simulink model "scars_example_appendix"  (R2019b)
settings: Solver=ode14x  StartTime=0.0  StopTime=300  FixedStep=0.1  RelTol=1e-3
libraries: scars_library x7
settings Model: Creator=asmialek  LastModifiedBy=asmialek
settings DataIOCC: ReturnWorkspaceOutputsName=scars_out

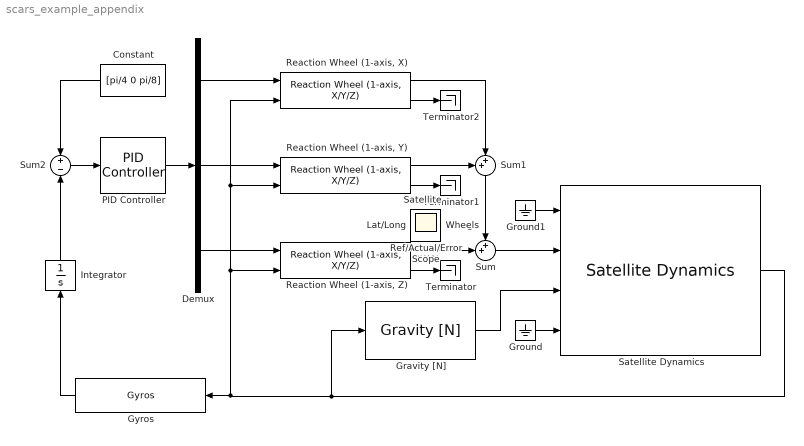
== system scars_example_appendix ==
  " Satellite Dynamics " : scars_library/Standard/ Satellite Dynamics   Parameter4=Keplerian Elements  epoch=0  mass=0  a=6356e3+400e3  e=0  incl=0  RA=0  w=0  TA=0  initEuler=[0 0 0]  initEulerRates=[0 0 0]  TA_copy=0  TA_copy_copy=400e3  TA_copy_copy_copy=[10 25]  TA_copy_copy_copy_copy=[10 25]  initEuler_copy=[0 0 0]  initEulerRates_copy=[0 0 0]  SSRTWFcnClass=[]
  Constant : Constant  Value=[pi/4 0 pi/8]
  Demux : Demux  Outputs=3
  Gravity [N] : scars_library/Environment/Gravity [N]  mass=1
  Ground : Ground
  Ground1 : Ground
  Gyros : scars_library/Sensors/Gyros  g_wn=14500  g_zeta=sqrt(2)/2  g_freq=10  g_bias=0  g_power=(2*pi*0.04/360)^2  g_max=deg2rad(75)  g_min=-deg2rad(75)
  Integrator : Integrator  InitialCondition=[0.76 2.32 1.71]
  PID Controller : scars_library/ Control Algorithms /PID Controller  Kp=700  Ki=0.01  Kd=1000  pid_sat_max=inf  pid_sat_min=-inf  pid_dz_max=0  pid_dz_min=0
  "Reaction Wheel (1-axis, X)" : scars_library/Actuators/Reaction Wheel (1-axis, X//Y//Z)  axis_switch=X  N=(1.5e-3)/0.5  R=12  J=300e-3  c=0  vel_max=6000*2*pi/60  torq_max=1.5e-3  i_max=0.5  rw_power=0  rw_freq=0.1
  "Reaction Wheel (1-axis, Y)" : scars_library/Actuators/Reaction Wheel (1-axis, X//Y//Z)  axis_switch=Y  N=(1.5e-3)/0.5  R=12  J=300e-3  c=0  vel_max=6000*2*pi/60  torq_max=1.5e-3  i_max=0.5  rw_power=0  rw_freq=0.1
  "Reaction Wheel (1-axis, Z)" : scars_library/Actuators/Reaction Wheel (1-axis, X//Y//Z)  axis_switch=Z  N=(1.5e-3)/0.5  R=12  J=300e-3  c=0  vel_max=6000*2*pi/60  torq_max=1.5e-3  i_max=0.5  rw_power=0  rw_freq=0.1
  Sum : Sum  Inputs=++|
  Sum1 : Sum  Inputs=++|
  Sum2 : Sum  Inputs=+|-
  Terminator : Terminator
  Terminator1 : Terminator
  Terminator2 : Terminator
  Lat/Long : Scope
  Omega : Scope
  RW Y : Scope
  Ref/Actual/Error : Scope
  Satellite : Scope
  Scope : Scope
  Wheels : Scope
  wires:
  Ground/1 -> " Satellite Dynamics "/4
  Gravity [N]/1 -> " Satellite Dynamics "/3
  " Satellite Dynamics "/1 -> Gravity [N]/1, "Reaction Wheel (1-axis, X)"/2, "Reaction Wheel (1-axis, Y)"/2, "Reaction Wheel (1-axis, Z)"/2, Gyros/1
  Ground1/1 -> " Satellite Dynamics "/1
  "Reaction Wheel (1-axis, Z)"/1 -> Sum/2
  "Reaction Wheel (1-axis, Z)"/2 -> Terminator/1
  "Reaction Wheel (1-axis, Y)"/2 -> Terminator1/1
  "Reaction Wheel (1-axis, X)"/2 -> Terminator2/1
  Sum/1 -> " Satellite Dynamics "/2
  "Reaction Wheel (1-axis, Y)"/1 -> Sum1/1
  Sum1/1 -> Sum/1
  "Reaction Wheel (1-axis, X)"/1 -> Sum1/2
  Sum2/1 -> PID Controller/1
  Gyros/1 -> Integrator/1
  Demux/1 -> "Reaction Wheel (1-axis, X)"/1
  Demux/2 -> "Reaction Wheel (1-axis, Y)"/1
  Demux/3 -> "Reaction Wheel (1-axis, Z)"/1
  Integrator/1 -> Sum2/2
  PID Controller/1 -> Demux/1
  Constant/1 -> Sum2/1
